simulink model "dbl_pendulum_model_verif"  (R2021b)
settings: Solver=VariableStepAuto  StartTime=0.0  StopTime=10.0  RelTol=1e-3
values from neighbouring files (symbols this model uses):
  b1 = 7.7210    (= 7.721)    [linearization_downdown.m]    (also in white_box_part1.m = truepars(9); white_box_part2.m = truepars(9))
  b2 = 2.337424773114795e-05    (= 2.33742477311e-05)    [linearization_downdown.m]    (also in white_box_part1.m = truepars(10); white_box_part2.m = truepars(10))
  c1 = -0.0320    (= -0.032)    [linearization_downdown.m]    (also in white_box_part1.m = truepars(5); white_box_part2.m = truepars(5))
  c2 = 0.053232610186913    (= 0.0532326101869)    [linearization_downdown.m]    (also in white_box_part1.m = truepars(6); white_box_part2.m = truepars(6))
  h = 0.001    [linearization_downdown.m]    (also in rotpentest.m = fugiboard('Open', 'pendulum1'); rotpentest3.m; white_box_part1.m; white_box_part2.m)
  I1 = 0.0888    [linearization_downdown.m]    (also in white_box_part1.m = truepars(7); white_box_part2.m = truepars(7))
  I2 = 9.5326e-05    [linearization_downdown.m]    (also in white_box_part1.m = truepars(8); white_box_part2.m = truepars(8))
  km = 53.049364666321930    (= 53.0493646663)    [linearization_downdown.m]    (also in white_box_part1.m = truepars(11); white_box_part2.m = truepars(11))
  l1 = 0.1    [linearization_downdown.m]    (also in white_box_part1.m = truepars(1); white_box_part2.m = truepars(1))
  l2 = 0.1    [linearization_downdown.m]    (also in white_box_part1.m = truepars(2); white_box_part2.m = truepars(2))
  m1 = 0.125    [linearization_downdown.m]    (also in white_box_part1.m = truepars(3); white_box_part2.m = truepars(3))
  m2 = 0.0493    [linearization_downdown.m]    (also in white_box_part1.m = truepars(4); white_box_part2.m = truepars(4))
  th1_0 = xbeam(1)    [white_box_part1.m]    (also in white_box_part2.m; white_box_verif.m)
  th2_0 = xpend(1)    [white_box_part1.m]    (also in white_box_part2.m; white_box_verif.m)
settings Model: Creator=MICHAEL-LT  LastModifiedBy=mfuser
settings DataIOCC: ReturnWorkspaceOutputs=off

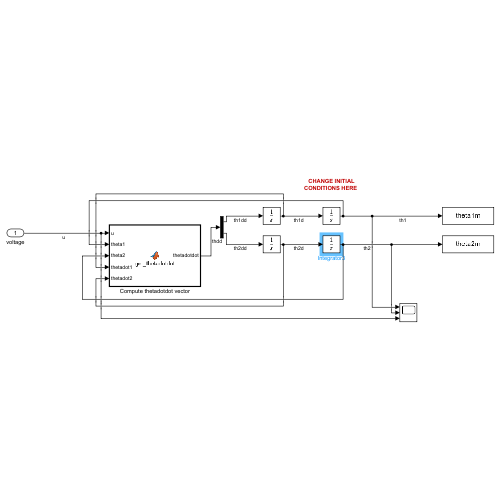
[thumbnail: Simulink's stored preview of the top-level diagram]
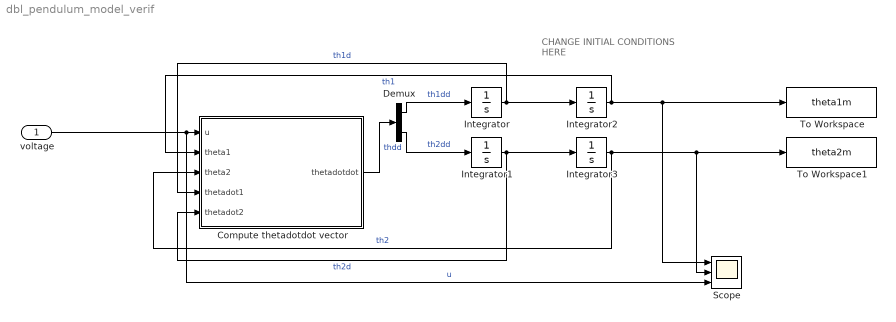
== system dbl_pendulum_model_verif ==
  note: CHANGE INITIAL CONDITIONS HERE
  voltage : Inport
  Compute thetadotdot vector : MATLAB Function  TreatAsAtomicUnit=on
  Demux : Demux  Outputs=2
  Integrator : Integrator
  Integrator1 : Integrator
  Integrator2 : Integrator  InitialCondition=th1_0
  Integrator3 : Integrator  InitialCondition=th2_0
  Scope : Scope  NumInputPorts=3
  To Workspace : ToWorkspace  VariableName=theta1m  SampleTime=h
  To Workspace1 : ToWorkspace  VariableName=theta2m  SampleTime=h
  wires:
  Demux/2 -> Integrator1/1  "th2dd"
  Demux/1 -> Integrator/1  "th1dd"
  Compute thetadotdot vector/1(thetadotdot) -> Demux/1  "thdd"
  Integrator1/1 -> Compute thetadotdot vector/5(thetadot2), Integrator3/1  "th2d"
  Integrator3/1 -> Scope/2, To Workspace1/1, Compute thetadotdot vector/3(theta2)  "th2"
  Integrator/1 -> Compute thetadotdot vector/4(thetadot1), Integrator2/1  "th1d"
  Integrator2/1 -> Scope/1, To Workspace/1, Compute thetadotdot vector/2(theta1)  "th1"
  voltage/1 -> Scope/3, Compute thetadotdot vector/1(u)  "u"

== matlab function dbl_pendulum_model_verif/Compute thetadotdot vector ==
  data: u input; thetadotdot output; theta1 input; theta2 input; thetadot1 input; thetadot2 input; l1 parameter; l2 parameter; m1 parameter; m2 parameter; c1 parameter; c2 parameter; I1 parameter; I2 parameter; b1 parameter; b2 parameter; km parameter
function thetadotdot  = get_thetadotdot(u, theta1, theta2, thetadot1, thetadot2, l1, l2, m1, m2, c1, c2, I1, I2, b1, b2, km)
%% Parameters (SI Units)
g = 9.81;
%% Variables of the model
th1 = theta1;
th2 = theta2;
th1d = thetadot1;
th2d = thetadot2;
thd_vec = [th1d ; th2d];
thetadotdot = [0 ; 0];
T_vec = [km*u ; 0];

%% Matrices of physical model
P1 = m1 * c1 * c1 + m2 * l1 * l1 + I1;
P2 = m2 * c2 * c2 + I2;
P3 = m2 * l1 * c2;
g1 = (m1 * c1 + m2 * l1) * g;
g2 = m2 * c2 * g;

M = [[P1 + P2 + 2*P3*cos(th2), P2 + P3 * cos(th2)]; [P2 + P3 * cos(th2) P2]];
C = [[b1 - P3 * th2d * sin(th2), -P3 * (th1d + th2d)*sin(th2)]; [P3 * th1d * sin(th2), b2]];
G = [- g1 * sin(th1) - g2 * sin(th1 + th2); - g2 * sin(th1 + th2)];

%% Compute output angular acceleration
M_inv = inv(M);
thetadotdot = M_inv*T_vec - M_inv*C*thd_vec - M_inv*G;
